simulink model "lab2"  (R2017b)
settings: Solver=ode45  StartTime=0.0  StopTime=1  RelTol=1e-3  EnableMultiTasking=on
values from neighbouring files (symbols this model uses):
  J = 0.71e-3    (= 0.00071)    [Lab2.m]
  ke = 0.33    [Lab2.m]
  km = ke    (= 0.33)    [Lab2.m]
  kp = 35    [Lab2.m]
  La = 14.28e-3    (= 0.01428)    [Lab2.m]
  Ra = 4.2    [Lab2.m]
  Rq = [1 -b-1 b]    [Lab2.m]
  S = [s2 s1 s0]    [Lab2.m]
  Tq = [(1+p1+p2)/K 0 0]    [Lab2.m]
  v = -0.2    [Lab2.m]
  vt = 0.6    [Lab2.m]
  w = 1    [Lab2.m]
settings Model: Creator=B014-5  LastModifiedBy=DNA
settings DataIOCC: LimitDataPoints=on  SaveFormat=Array
settings OptimizationCC: LifeSpan=inf
settings DebuggingCC: SFUnexpectedBacktrackingDiag=warning  SFNoUnconditionalDefaultTransitionDiag=warning  SFExecutionAtInitializationDiag=none
settings HardwareCC: ProdBitPerPointer=32  ProdBitPerSizeT=32  ProdBitPerPtrDiffT=32  ProdLargestAtomicFloat=None  ProdIntDivRoundTo=Undefined  ProdEndianess=Unspecified  ProdWordSize=32  ProdHWDeviceType=32-bit Generic
settings ModelReferenceCC: PropagateSignalLabelsOutOfModel=off
settings CodeAppCC: StateflowObjectComments=on
settings GRTTargetCC: TargetLangStandard=C89/C90 (ANSI)  GeneratePreprocessorConditionals=Disable all
settings ConfigComp: CovMetricSettings=dw  CovHtmlReporting=on  CovSaveCumulativeToWorkspaceVar=on  CovSaveSingleToWorkspaceVar=on  CovExternalEMLEnable=off

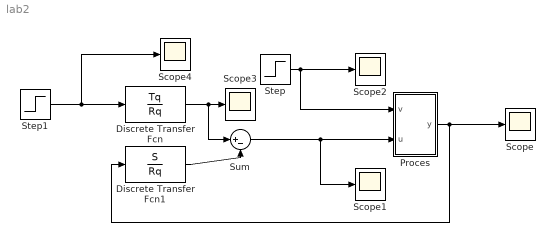
== system lab2 ==
  Discrete Transfer Fcn : DiscreteTransferFcn  Numerator=Tq  Denominator=Rq
  Discrete Transfer Fcn1 : DiscreteTransferFcn  Numerator=S  Denominator=Rq
  Proces : Subsystem
  Scope{,1..4} (5 alike) : Scope
  Step : Step  Time=vt  After=v  SampleTime=0
  Step1 : Step  Time=0  After=w  SampleTime=0
  Sum : Sum  Inputs=|+-
  wires:
  Step/1 -> Scope2/1, Proces/1(v)
  Discrete Transfer Fcn1/1 -> Sum/2
  Sum/1 -> Scope1/1, Proces/2(u)
  Proces/1(y) -> Scope/1, Discrete Transfer Fcn1/1
  Discrete Transfer Fcn/1 -> Scope3/1, Sum/1
  Step1/1 -> Scope4/1, Discrete Transfer Fcn/1

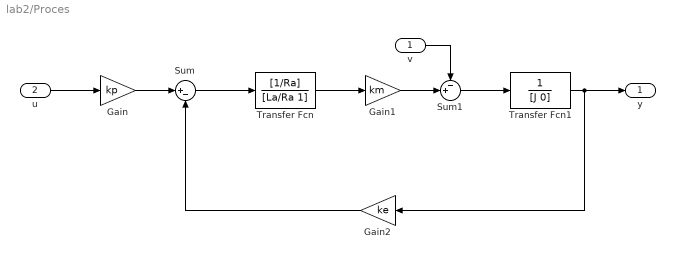
== system lab2/Proces ==
  v : Inport
  u : Inport  Port=2
  Gain : Gain  Gain=kp
  Gain1 : Gain  Gain=km
  Gain2 : Gain  Gain=ke
  Sum : Sum  Inputs=|+-
  Sum1 : Sum  Inputs=-+|
  Transfer Fcn : TransferFcn  Numerator=[1/Ra]  Denominator=[La/Ra 1]
  Transfer Fcn1 : TransferFcn  Denominator=[J 0]
  y : Outport
  wires:
  v/1 -> Sum1/1
  Gain/1 -> Sum/1
  Transfer Fcn1/1 -> y/1, Gain2/1
  Sum1/1 -> Transfer Fcn1/1
  Sum/1 -> Transfer Fcn/1
  Gain2/1 -> Sum/2
  u/1 -> Gain/1
  Gain1/1 -> Sum1/2
  Transfer Fcn/1 -> Gain1/1
